simulink model "ImuCalibrator3Pass"  (R2018a)
settings: Solver=FixedStepDiscrete  StartTime=0.0  StopTime=inf  FixedStep=1/Fss  RelTol=1e-3
PreLoadFcn:
  | busDef
  | Fss = 1125;
  | Fss = 2100;
InitFcn:
  | modelDef = getModelDef(true);
undefined symbols (not defined in the file or in its folder): df, dw, Ggyr, Macc, Mgyr, numStates
libraries: simulink x15, vrlib x15, dspsigops x6, dspindex x6, dspinverses x6, dspstat3 x3, simulink_extras x3, dspmtrx3 x3, dspsrcs4 x3, dspmathops x3, dspswit3 x1
(part 4 of 4)

== matlab function ImuCalibrator3Pass/saveCalQuality ==
  data: fileReadError input; limits input; numStills input; firstPassCorrections input Bus: corrections; secondPassCorrections input Bus: corrections; thirdPassCorrections input Bus: corrections; calPass output
function calPass = saveCalQuality(fileReadError, limits, numStills, firstPassCorrections, secondPassCorrections, thirdPassCorrections)

fid = fopen('imuCalQuality.txt', 'w');
calPass = true;

if fileReadError
    calPass = false;
    fprintf(fid, 'FAIL :  imudata.txt file not read\n');
end

if numStills < 6
    calPass = false;
    fprintf(fid, 'FAIL : insufficient still times detected (possibly noisy sensor)\n');
end
fprintf(fid, 'Num stills over 5s duration: %d\n\n', int8(numStills));

% first pass corrections
fprintf(fid, '**********************  FIRST PASS ****************************\n');
gyroBiasLim = limits(1,1); %3*0.01;
gyroSfLim = limits(1,2);  %3*0.01;
gyroMaLim = limits(1,3);  %3*0.01;
accelBiasLim = limits(1,4);  %3*40*9.8/1000;
accelSfLim = limits(1,5);  %3*0.01;
accelMaLim = limits(1,6);  %3*0.01;
corrections = firstPassCorrections;
gyroBiases = [ corrections.dw(1) corrections.dw(2) corrections.dw(3)];
gyroSf = [corrections.Mgyr(1,1) corrections.Mgyr(2,2) corrections.Mgyr(3,3)];
gyroMa = [corrections.Mgyr(1,2) corrections.Mgyr(1,3) corrections.Mgyr(2,1) corrections.Mgyr(2,3) corrections.Mgyr(3,1) corrections.Mgyr(3,2)];
accelBiases = [ corrections.df(1) corrections.df(2) corrections.df(3)];
accelSf = [corrections.Macc(1,1) corrections.Macc(2,2) corrections.Macc(3,3)];
accelMa = [corrections.Macc(1,2) corrections.Macc(1,3) corrections.Macc(2,1) corrections.Macc(2,3) corrections.Macc(3,1) corrections.Macc(3,2)];



fprintf(fid, 'Gyro biases (deg/hr):\n');
rps2dph = 180/pi*3600;
calPass = calPass & printTriadResults(fid, gyroBiases*rps2dph, gyroBiasLim*rps2dph);

fprintf(fid, 'Gyro scale factors:\n');
calPass = calPass & printTriadResults(fid, gyroSf, gyroSfLim);

fprintf(fid, 'Gyro misalignments:\n');
calPass = calPass & printTriadResults(fid, gyroMa, gyroMaLim);

fprintf(fid, 'Accel biases (mg):\n');
mpss2mg = 1000/9.8;
calPass = calPass & printTriadResults(fid, accelBiases*mpss2mg, accelBiasLim*mpss2mg);

fprintf(fid, 'Accel scale factors:\n');
calPass = calPass & printTriadResults(fid, accelSf, accelSfLim);

fprintf(fid, 'Accel misalignments:\n');
calPass = calPass & printTriadResults(fid, accelMa, accelMaLim);



% second pass corrections
fprintf(fid, '**********************  SECOND PASS ****************************\n');
gyroBiasLim = limits(2,1);  %0.001;
gyroSfLim = limits(2,2);  %2e-3;
gyroMaLim = limits(2,3);  %2e-3;
accelBiasLim = limits(2,4);  %2 * 9.8/1000;
accelSfLim = limits(2,5);  %0.001;
accelMaLim = limits(2,6);  %0.003;
corrections = secondPassCorrections;
gyroBiases = [ corrections.dw(1) corrections.dw(2) corrections.dw(3)];
gyroSf = [corrections.Mgyr(1,1) corrections.Mgyr(2,2) corrections.Mgyr(3,3)];
gyroMa = [corrections.Mgyr(1,2) corrections.Mgyr(1,3) corrections.Mgyr(2,1) corrections.Mgyr(2,3) corrections.Mgyr(3,1) corrections.Mgyr(3,2)];
accelBiases = [ corrections.df(1) corrections.df(2) corrections.df(3)];
accelSf = [corrections.Macc(1,1) corrections.Macc(2,2) corrections.Macc(3,3)];
accelMa = [corrections.Macc(1,2) corrections.Macc(1,3) corrections.Macc(2,1) corrections.Macc(2,3) corrections.Macc(3,1) corrections.Macc(3,2)];

fprintf(fid, 'Gyro biases (deg/hr):\n');
rps2dph = 180/pi*3600;
calPass = calPass & printTriadResults(fid, gyroBiases*rps2dph, gyroBiasLim*rps2dph);

fprintf(fid, 'Gyro scale factors:\n');
calPass = calPass & printTriadResults(fid, gyroSf, gyroSfLim);

fprintf(fid, 'Gyro misalignments:\n');
calPass = calPass & printTriadResults(fid, gyroMa, gyroMaLim);

fprintf(fid, 'Accel biases (mg):\n');
mpss2mg = 1000/9.8;
calPass = calPass & printTriadResults(fid, accelBiases*mpss2mg, accelBiasLim*mpss2mg);

fprintf(fid, 'Accel scale factors:\n');
calPass = calPass & printTriadResults(fid, accelSf, accelSfLim);

fprintf(fid, 'Accel misalignments:\n');
calPass = calPass & printTriadResults(fid, accelMa, accelMaLim);



% third pass corrections
fprintf(fid, '**********************  THIRD PASS ****************************\n');
gyroBiasLim = limits(3,1); %3e-4;
gyroSfLim = limits(3,2); %2e-3;
gyroMaLim = limits(3,3); %2e-3;
accelBiasLim = limits(3,4); %0.3 * 9.8/1000;
accelSfLim = limits(3,5); %0.0003;
accelMaLim = limits(3,6); %0.0015;
corrections = thirdPassCorrections;
gyroBiases = [ corrections.dw(1) corrections.dw(2) corrections.dw(3)];
gyroSf = [corrections.Mgyr(1,1) corrections.Mgyr(2,2) corrections.Mgyr(3,3)];
gyroMa = [corrections.Mgyr(1,2) corrections.Mgyr(1,3) corrections.Mgyr(2,1) corrections.Mgyr(2,3) corrections.Mgyr(3,1) corrections.Mgyr(3,2)];
accelBiases = [ corrections.df(1) corrections.df(2) corrections.df(3)];
accelSf = [corrections.Macc(1,1) corrections.Macc(2,2) corrections.Macc(3,3)];
accelMa = [corrections.Macc(1,2) corrections.Macc(1,3) corrections.Macc(2,1) corrections.Macc(2,3) corrections.Macc(3,1) corrections.Macc(3,2)];

fprintf(fid, 'Gyro biases (deg/hr):\n');
rps2dph = 180/pi*3600;
calPass = calPass & printTriadResults(fid, gyroBiases*rps2dph, gyroBiasLim*rps2dph);

fprintf(fid, 'Gyro scale factors:\n');
calPass = calPass & printTriadResults(fid, gyroSf, gyroSfLim);

fprintf(fid, 'Gyro misalignments:\n');
calPass = calPass & printTriadResults(fid, gyroMa, gyroMaLim);

fprintf(fid, 'Accel biases (mg):\n');
mpss2mg = 1000/9.8;
calPass = calPass & printTriadResults(fid, accelBiases*mpss2mg, accelBiasLim*mpss2mg);

fprintf(fid, 'Accel scale factors:\n');
calPass = calPass & printTriadResults(fid, accelSf, accelSfLim);

fprintf(fid, 'Accel misalignments:\n');
calPass = calPass & printTriadResults(fid, accelMa, accelMaLim);






fclose(fid);

calPass = true;



function pass = printTriadResults(fid, values, limit)
for i=1:length(values)
    fprintf(fid, '%10.6f ', values(i)); 
end
fprintf(fid, '(limit %f) \n', limit);
pctLim = max(abs(values))/limit * 100;
if  pctLim <= 100 
    fprintf(fid, 'PASS (%4.1f %% of limit)\n\n', pctLim); pass = true;
else
    fprintf(fid, 'FAIL (%4.1f %% of limit)\n\n', pctLim);  pass = false;
end

== matlab function ImuCalibrator3Pass/MATLAB Function1 ==
  data: gyroCalBiases output; gyroCalMatrix output; dw input; Mgyr input; df input; Macc input; Ggyr input; accelCalBiases output; accelCalMatrix output; gyroGsensMatrix output
function [gyroCalBiases, gyroCalMatrix, accelCalBiases, accelCalMatrix,  gyroGsensMatrix] = updateCal(dw, Mgyr, df, Macc, Ggyr)

    

    gyroCalBiases =  (eye(3)+Mgyr)*dw;
    gyroGsensMatrix = (eye(3)+Mgyr)*Ggyr;
    gyroCalMatrix = inv(eye(3) + Mgyr);

    accelCalBiases =  df + Macc*df;
    accelCalMatrix =inv(eye(3) + Macc);

== matlab function ImuCalibrator3Pass/MATLAB Function2 ==
  data: gyroCalBiases output; gyroCalMatrix output; dw input; Mgyr input; df input; Macc input; Ggyr input; gyroCalBiases input; gyroCalMatrix input; accelCalBiases input; accelCalMatrix input; gyroGsensMatrix input; accelCalBiases output; accelCalMatrix output; gyroGsensMatrix output
function [gyroCalBiases, gyroCalMatrix, accelCalBiases, accelCalMatrix,  gyroGsensMatrix] = updateCal2(dw, Mgyr, df, Macc, Ggyr, gyroCalBiases, gyroCalMatrix, accelCalBiases, accelCalMatrix,  gyroGsensMatrix)

    gyroCalBiases = gyroCalBiases + (eye(3)+Mgyr)*dw;
    gyroGsensMatrix = gyroGsensMatrix + (eye(3)+Mgyr)*Ggyr;
    gyroCalMatrix = inv(eye(3) + Mgyr) * gyroCalMatrix;

    accelCalBiases = accelCalBiases + df + Macc*df;
    accelCalMatrix =inv(eye(3) + Macc) * accelCalMatrix;

== matlab function ImuCalibrator3Pass/firstPass/MATLAB Function1 ==
  data: datarow output; EOF output
function [datarow, EOF] = readLineAscii()

persistent data data2 nrows row

if isempty(data)
    % row format = # SeqID, DeviceID, timestamp (sec), gyroXYZ (rad/sec), accelXYZ (m/s^2), temperature (degC)
    coder.varsize('data', [500000, 10], [1 0]);  % ten columns,  up to 200k rows
    data = load('imudata.txt', '-ascii'); 
    
    validTimestamp = data(:,3) > 0.001;
    data2 = data(validTimestamp, [4 5 6 7 8 9 3]); % select just the useful columns and rows
    nrows = size(data2, 1);
    row = 2;  % skip the first row since we need delta-t's

end

datarow = data2(row,:)';
datarow(7) = data2(row,7) - data2(row-1,7); % calculate Delta-t

EOF = row >= nrows;
row = row + 1;

== matlab function ImuCalibrator3Pass/secondPass/AINS/INS/MATLAB Function2 ==
  data: Cbn input; Cbn_new output; w input; dt input
function Cbn_new = update_dcm(Cbn, w, dt)

% Update attitude according to TW p.312 approximated to sixth order

rot=w*dt;
rot_norm=norm(rot);
sr_a=1-(rot_norm^2/6)+(rot_norm^4/120);
sr_b=(1/2)-(rot_norm^2/24)+(rot_norm^4/720);
mx_a=eye(3)+sr_a*skew(rot)+sr_b*skew(rot)*skew(rot);

Cbn_new=Cbn*mx_a;


function res=skew(inp_vr)
res=[0 			-inp_vr(3)	inp_vr(2); ...
     inp_vr(3)	0			-inp_vr(1);...
	 -inp_vr(2)	inp_vr(1)	0];

== matlab function ImuCalibrator3Pass/secondPass/AINS/MATLAB Function ==
  data: w input; stilltime output; f input; Dt input; favgs output; wavgs output
function [stilltime, favgs, wavgs] = update_stilltime(w, f, Dt)

persistent stillt wavg favg stillcycles wsigmas fsigmas;

if isempty(wavg)
    stillt = 0;
    stillcycles = 0;
    wavg = w;
    favg = f;
    wsigmas = 0.02*[1;1;1];%%0.01*[1;1;1];
    fsigmas = 0.4*[1;1;1];%0.2*[1;1;1];
end

if all(abs(f-favg) < 3*fsigmas) && all(abs(w-wavg) < 3*wsigmas)  % increment the stilltimes
    stillt = stillt + Dt;
    stillcycles = stillcycles + 1;
%     % simple recursive mean (weighting all the samples equally):
%     wavg = ((stillcycles-1)*wavg + w)/stillcycles;
%     favg = ((stillcycles-1)*favg + f)/stillcycles;

%     % recursive mean with each sample weighted by the stillcycles when it came in:
%     wavg = ((stillcycles-1)*wavg + 2*w)/(stillcycles+1);
%     favg = ((stillcycles-1)*favg + 2*f)/(stillcycles+1);

    % start with stilltime weighting and switch back to simple recursive mean after 1 second to reduce noise:
    if stillt < 1
        wavg = ((stillcycles-1)*wavg + 2*w)/(stillcycles+1);
        favg = ((stillcycles-1)*favg + 2*f)/(stillcycles+1);
    else
        wavg = ((stillcycles-1)*wavg + w)/stillcycles;
        favg = ((stillcycles-1)*favg + f)/stillcycles;
    end        
else  %reset stilltime
    stillt = 0;
    stillcycles = 0;
    wavg = w;
    favg = f;
end    

stilltime = stillt;
favgs = favg;
wavgs = wavg;

== matlab function ImuCalibrator3Pass/secondPass/AINS/compass meas update/MATLAB Function1 ==
  data: S output; P input; K output; H input; R input
function [S,K] = calcKalmanGain(P, H, R)

PHT = P*H';
S = H*PHT + R;
K = PHT/S;

== matlab function ImuCalibrator3Pass/secondPass/AINS/compass meas update/MATLAB Function3 ==
  data: P input; Pplus output; K input; H input; R input; IminKH output
function [Pplus, IminKH] = josephCovarianceUpdate(P, K, H, R)

IminKH = eye(size(P)) - K*H;
Pplus = IminKH*P*IminKH' + K*R*K';

== matlab function ImuCalibrator3Pass/secondPass/AINS/compass meas update/update the Cbn with the errors/MATLAB Function ==
  data: inp_vr input; res output
function res=skew(inp_vr)
res=[0 			-inp_vr(3)	inp_vr(2); ...
     inp_vr(3)	0			-inp_vr(1);...
	 -inp_vr(2)	inp_vr(1)	0];

== matlab function ImuCalibrator3Pass/firstPass/AINS/gravity meas update/MATLAB Function2 ==
  data: inp_vr input; res output
function res=skew(inp_vr)
res=[0 			-inp_vr(3)	inp_vr(2); ...
     inp_vr(3)	0			-inp_vr(1);...
	 -inp_vr(2)	inp_vr(1)	0];

== matlab function ImuCalibrator3Pass/firstPass/AINS/compass meas update/MATLAB Function1 ==
  data: S output; P input; K output; H input; R input
function [S,K] = calcKalmanGain(P, H, R)

PHT = P*H';
S = H*PHT + R;
K = PHT/S;

== matlab function ImuCalibrator3Pass/secondPass/AINS/gravity meas update/MATLAB Function1 ==
  data: S output; P input; K output; H input; R input
function [S,K] = calcKalmanGain(P, H, R)

PHT = P*H';
S = H*PHT + R;
K = PHT/S;

== matlab function ImuCalibrator3Pass/secondPass/AINS/gravity meas update/MATLAB Function2 ==
  data: inp_vr input; res output
function res=skew(inp_vr)
res=[0 			-inp_vr(3)	inp_vr(2); ...
     inp_vr(3)	0			-inp_vr(1);...
	 -inp_vr(2)	inp_vr(1)	0];

== matlab function ImuCalibrator3Pass/secondPass/AINS/gravity meas update/MATLAB Function3 ==
  data: P input; Pplus output; K input; H input; R input; IminKH output
function [Pplus, IminKH] = josephCovarianceUpdate(P, K, H, R)

IminKH = eye(size(P)) - K*H;
Pplus = IminKH*P*IminKH' + K*R*K';

== matlab function ImuCalibrator3Pass/secondPass/AINS/gravity meas update/update the Cbn and b_g with the errors/MATLAB Function ==
  data: inp_vr input; res output
function res=skew(inp_vr)
res=[0 			-inp_vr(3)	inp_vr(2); ...
     inp_vr(3)	0			-inp_vr(1);...
	 -inp_vr(2)	inp_vr(1)	0];

== matlab function ImuCalibrator3Pass/secondPass/AINS/initialize states and covariances/set P/MATLAB Function1 ==
  data: initialRotUncert input; initialPosUncert input; initialVelUncert input; P0 output size=[modelDef.numStates, modelDef.numStates]; modelDef parameter; imuPar parameter
function P0  = calculate_P0(initialRotUncert, initialPosUncert, initialVelUncert, modelDef, imuPar)

% order of the states:
% 1:3   phi
% 4:6   dw
% 7:9   dr
% 10:12 dv
% 13:15 df  (if modelDef.trackAccelBiases)
% 16:24 dM_gyro in column-major order (if modelDef.trackGyroSfma)
% 25:33 dM_accel in column-major order (if modelDef.trackAccelSfma)
% 34:42 dG_gyro in column-major order (if modelDef.trackGyroGsens)

P0 = zeros(modelDef.numStates, modelDef.numStates);

P0(1:3, 1:3) = diag(initialRotUncert.^2);
P0(4:6, 4:6) = eye(3)*(imuPar.gyroBiasUncert.^2);
P0(7:9, 7:9) = diag(initialPosUncert.^2);
P0(10:12, 10:12) = diag(initialVelUncert.^2);


if modelDef.trackAccelBiases
    P0(13:15, 13:15) = eye(3)*(imuPar.accelBiasUncert.^2);
end

if modelDef.trackGyroSfma  
    vec9 = ones(9,1)*imuPar.gyroAlignUncert^2;
    vec9([1 5 9]) = imuPar.gyroScaleUncert^2;
    P0(16:24, 16:24) = diag(vec9);
end

if modelDef.trackAccelSfma  % propagate dM_accel to dv
    vec9 = ones(9,1)*imuPar.accelAlignUncert^2;
    vec9([1 5 9]) = imuPar.accelScaleUncert^2;
    if modelDef.accelDefinesExtrinsics
        vec9([4 7]) = 0.0001^2; % x accel has no misalignment so picks up no component of y or z accelerations
        vec9(8) = 0.0001^2;  % y accel has no tilt out of xy plane, so picks up no component of z acceleration
    end
    P0(25:33, 25:33) = diag(vec9);
end

if modelDef.trackGyroGsens
    vec9 = ones(9,1)*imuPar.gyroGsensUncert^2;
    P0(34:42, 34:42) = diag(vec9);
end

== matlab function ImuCalibrator3Pass/firstPass/AINS/compass meas update/MATLAB Function3 ==
  data: P input; Pplus output; K input; H input; R input; IminKH output
function [Pplus, IminKH] = josephCovarianceUpdate(P, K, H, R)

IminKH = eye(size(P)) - K*H;
Pplus = IminKH*P*IminKH' + K*R*K';

== matlab function ImuCalibrator3Pass/secondPass/AINS/report output/MATLAB Function1 ==
  data: Cbn input; quat output size=[4,1]
function quat=dcm2quat(Cbn)

%dcm (Cba) to quaternion (qba)
%Cba:B to A transformation matrix
%qba:B to A quaternion

%Implementation of savage(3-47)


tr=Cbn(1,1)+Cbn(2,2)+Cbn(3,3);
Pa=1+tr;
Pb=1+2*Cbn(1,1)-tr;
Pc=1+2*Cbn(2,2)-tr;
Pd=1+2*Cbn(3,3)-tr;

quat=zeros(4,1);
if (Pa>=Pb && Pa>=Pc && Pa>=Pd)
    quat(1)=0.5*sqrt(Pa);
    quat(2)=(Cbn(3,2)-Cbn(2,3))/4/quat(1);
    quat(3)=(Cbn(1,3)-Cbn(3,1))/4/quat(1);
    quat(4)=(Cbn(2,1)-Cbn(1,2))/4/quat(1);
elseif (Pb>=Pc && Pb>=Pd)
    quat(2)=0.5*sqrt(Pb);
    quat(3)=(Cbn(2,1)+Cbn(1,2))/4/quat(2);
    quat(4)=(Cbn(1,3)+Cbn(3,1))/4/quat(2);
    quat(1)=(Cbn(3,2)-Cbn(2,3))/4/quat(2);
elseif (Pc>=Pd)
    quat(3)=0.5*sqrt(Pc);
    quat(4)=(Cbn(3,2)+Cbn(2,3))/4/quat(3);
    quat(1)=(Cbn(1,3)-Cbn(3,1))/4/quat(3);
    quat(2)=(Cbn(2,1)+Cbn(1,2))/4/quat(3);
else
    quat(4)=0.5*sqrt(Pd);
    quat(1)=(Cbn(2,1)-Cbn(1,2))/4/quat(4);
    quat(2)=(Cbn(1,3)+Cbn(3,1))/4/quat(4);
    quat(3)=(Cbn(3,2)+Cbn(2,3))/4/quat(4);
end

if (quat(1)<=0)
    quat=-quat;
end

== matlab function ImuCalibrator3Pass/secondPass/AINS/report output/MATLAB Function3 ==
  data: Cbn input; eul output size=[3,1]
function eul = dcm2euler(Cbn)

%DCM is Cbn (transforms vectors from b to n)
%eul defined as zyx sequence (yaw,pitch,roll),  but listed in
%roll,pitch,yaw order


pitch=asin(-Cbn(3,1));  %pitch is assumed to be [-pi pi]. singular at pi. use ad-hoc methods to remedy this deficiency
roll=atan2(Cbn(3,2), Cbn(3,3));
heading = atan2(Cbn(2,1), Cbn(1,1));
eul=[roll;pitch;heading];

== matlab function ImuCalibrator3Pass/firstPass/AINS/compass meas update/update the Cbn with the errors/MATLAB Function ==
  data: inp_vr input; res output
function res=skew(inp_vr)
res=[0 			-inp_vr(3)	inp_vr(2); ...
     inp_vr(3)	0			-inp_vr(1);...
	 -inp_vr(2)	inp_vr(1)	0];

== matlab function ImuCalibrator3Pass/secondPass/AINS/time update/MATLAB Function ==
  data: omega input; Q output size=[modelDef.numStates, modelDef.numStates]; f_ib input; Dt input; Cbn input; modelDef parameter; imuPar parameter
function Q  = calculate_Q(omega, f_ib, Dt, Cbn, modelDef, imuPar)

% order of the states:
% 1:3   phi
% 4:6   dw
% 7:9   dr
% 10:12 dv
% 13:15 df  (if modelDef.trackAccelBiases)
% 16:24 dM_gyro in column-major order (if modelDef.trackGyroSfma)
% 25:33 dM_accel in column-major order (if modelDef.trackAccelSfma)

Q = zeros(modelDef.numStates, modelDef.numStates);

omega = reshape(omega,3,1); 
f_ib = reshape(f_ib, 3,1);

Qphi = diag((imuPar.gyroArwRadPerRtSec^2)*[Dt Dt Dt]);  
Qdw = diag((imuPar.gyroBrwRadPerSecPerRtSec^2)*[Dt Dt Dt]);
Qdv = diag((imuPar.accelVrwMetersPerSecPerRtSec^2)*[Dt Dt Dt]);
Qdf = diag((imuPar.accelBrwMetersPerSec2PerRtSec^2)*[Dt Dt Dt]);


%bump up Q for unmodelled states
if ~modelDef.trackGyroSfma % gyro scale factor and misalignment not tracked
   gyroSfSigmaBod = imuPar.gyroScaleUncert*omega;
   gyroMaSigmaBod = imuPar.gyroAlignUncert*sqrt(omega'*omega*[1 1 1]-omega'.*omega');   
   QgyroMa = Cbn*diag(gyroMaSigmaBod.^2)*Cbn'*Dt; 
   QgyroSf = Cbn*diag(gyroSfSigmaBod.^2)*Cbn'*Dt; 
   Qphi = Qphi + QgyroMa + QgyroSf;   
end

if ~modelDef.trackGyroGsens %  gyro g sensitivity not tracked 
   gGsensSigmaBod = imuPar.gyroGsensUncert*sqrt(f_ib'*f_ib*[1 1 1]-f_ib'.*f_ib');   
   QgGsens = Cbn*diag(gGsensSigmaBod.^2)*Cbn'*Dt; 
   Qphi = Qphi + QgGsens;   
end

if ~modelDef.trackAccelSfma  % accel scale factor and misalignment not tracked
   accelSfSigmaBod = imuPar.accelScaleUncert*f_ib;
   accelMaSigmaBod = imuPar.accelAlignUncert*sqrt(f_ib'*f_ib*[1 1 1]-f_ib'.*f_ib');   
   QaccelMa = Cbn*diag(accelMaSigmaBod.^2)*Cbn'*Dt; 
   QaccelSf = Cbn*diag(accelSfSigmaBod.^2)*Cbn'*Dt; 
   Qdv = Qdv + QaccelMa + QaccelSf;   
end

Q(1:3, 1:3) = Qphi;
Q(4:6, 4:6) = Qdw;
Q(10:12, 10:12) = Qdv;
Q(13:15, 13:15) = Qdf;

== matlab function ImuCalibrator3Pass/secondPass/AINS/time update/MATLAB Function1 ==
  data: imuPar output Bus: imuPar
function imuPar = imuPar

imuPar.gyroArwDegPerRtHr = 0.25;
imuPar.gyroArwRadPerRtSec = imuPar.gyroArwDegPerRtHr * pi/180/60;
imuPar.gyroBrwDegPerHrPerRtHr = 0;
imuPar.gyroBrwRadPerSecPerRtSec = imuPar.gyroBrwDegPerHrPerRtHr * pi/180/3600/60;
imuPar.gyroScaleUncertainty = 0.001;
imuPar.gyroAlignUncertainty = 0.01;
imuPar.gyroGsensUncertainty = 0.001;

== matlab function ImuCalibrator3Pass/secondPass/AINS/time update/MATLAB Function2 ==
  settings: updateMethod=DISCRETE  sampleTime=inf
  data: modelDef output Bus: modelDef; numStates input
function modelDef = modelDef(numStates)

modelDef.trackAccelBiases = true;
modelDef.trackAccelSfma = true;
modelDef.trackGyroSfma = true;
modelDef.trackGyroGsens = false;

modelDef.numStates = numStates;

== matlab function ImuCalibrator3Pass/secondPass/AINS/time update/MATLAB Function3 ==
  data: omega input; Phi output size=[modelDef.numStates, modelDef.numStates]; fbod input; Dt input; Cbn input; modelDef parameter
function Phi  = calculate_Phi(omega, fbod, Dt, Cbn, modelDef)

% order of the states:
% 1:3   phi
% 4:6   dw
% 7:9   dr
% 10:12 dv
% 13:15 df  (if modelDef.trackAccelBiases)
% 16:24 dM_gyro in column-major order (if modelDef.trackGyroSfma)
% 25:33 dM_accel in column-major order (if modelDef.trackAccelSfma)
% 34:42 dG_gyro in column-major order (if modelDef.trackGyroGsens)

Phi = eye(modelDef.numStates);

DtC = Dt*Cbn;

Phi(1:3,4:6) = -DtC;  % propagate dw to phi
Phi(7:9, 10:12) = Dt*eye(3);  % propagate dv to dr
Phi(10:12, 1:3) = Dt*skew(Cbn*fbod);  % propagate phi to dv

if modelDef.trackAccelBiases
    Phi(10:12, 13:15) = DtC;   % propagate df to dv
end

if modelDef.trackGyroSfma  % propagate dM_gyro to phi
    Phi(1:3, 16:18) = -DtC*omega(1);
    Phi(1:3, 19:21) = -DtC*omega(2);
    Phi(1:3, 22:24) = -DtC*omega(3);
end

if modelDef.trackAccelSfma  % propagate dM_accel to dv
    Phi(10:12, 25:27) = DtC*fbod(1);
    Phi(10:12, 28:30) = DtC*fbod(2);
    Phi(10:12, 31:33) = DtC*fbod(3);
end

if modelDef.trackGyroGsens  % propagate dG_gyro to phi
    Phi(1:3, 34:36) = -DtC*fbod(1);
    Phi(1:3, 37:39) = -DtC*fbod(2);
    Phi(1:3, 40:42) = -DtC*fbod(3);
end


function res=skew(inp_vr)
res=[0 			-inp_vr(3)	inp_vr(2); ...
     inp_vr(3)	0			-inp_vr(1);...
	 -inp_vr(2)	inp_vr(1)	0];

== matlab function ImuCalibrator3Pass/secondPass/AINS/zero velocity update/MATLAB Function1 ==
  data: S output; P input; K output; H input; R input
function [S,K] = calcKalmanGain(P, H, R)

PHT = P*H';
S = H*PHT + R;
K = PHT/S;

== matlab function ImuCalibrator3Pass/secondPass/AINS/zero velocity update/MATLAB Function3 ==
  data: P input; Pplus output; K input; H input; R input; IminKH output
function [Pplus, IminKH] = josephCovarianceUpdate(P, K, H, R)

IminKH = eye(size(P)) - K*H;
Pplus = IminKH*P*IminKH' + K*R*K';

== matlab function ImuCalibrator3Pass/secondPass/AINS/zero velocity update/update the underlying states/MATLAB Function ==
  data: inp_vr input; res output
function res=skew(inp_vr)
res=[0 			-inp_vr(3)	inp_vr(2); ...
     inp_vr(3)	0			-inp_vr(1);...
	 -inp_vr(2)	inp_vr(1)	0];

== matlab function ImuCalibrator3Pass/secondPass/printTime/MATLAB Function ==
  data: u input
function  printTime(u)
%#codegen

% using fileId = 1  only generates a printf in the generated code
% fileId = 2 also causes prints in the matlab console

fprintf(2, "\r 2nd pass: %f sec", u);

== matlab function ImuCalibrator3Pass/thirdPass/AINS/INS/MATLAB Function2 ==
  data: Cbn input; Cbn_new output; w input; dt input
function Cbn_new = update_dcm(Cbn, w, dt)

% Update attitude according to TW p.312 approximated to sixth order

rot=w*dt;
rot_norm=norm(rot);
sr_a=1-(rot_norm^2/6)+(rot_norm^4/120);
sr_b=(1/2)-(rot_norm^2/24)+(rot_norm^4/720);
mx_a=eye(3)+sr_a*skew(rot)+sr_b*skew(rot)*skew(rot);

Cbn_new=Cbn*mx_a;


function res=skew(inp_vr)
res=[0 			-inp_vr(3)	inp_vr(2); ...
     inp_vr(3)	0			-inp_vr(1);...
	 -inp_vr(2)	inp_vr(1)	0];

== matlab function ImuCalibrator3Pass/thirdPass/AINS/MATLAB Function ==
  data: w input; stilltime output; f input; Dt input; favgs output; wavgs output
function [stilltime, favgs, wavgs] = update_stilltime(w, f, Dt)

persistent stillt wavg favg stillcycles wsigmas fsigmas;

if isempty(wavg)
    stillt = 0;
    stillcycles = 0;
    wavg = w;
    favg = f;
    wsigmas = 0.02*[1;1;1];%%0.01*[1;1;1];
    fsigmas = 0.4*[1;1;1];%0.2*[1;1;1];
end

if all(abs(f-favg) < 3*fsigmas) && all(abs(w-wavg) < 3*wsigmas)  % increment the stilltimes
    stillt = stillt + Dt;
    stillcycles = stillcycles + 1;
%     % simple recursive mean (weighting all the samples equally):
%     wavg = ((stillcycles-1)*wavg + w)/stillcycles;
%     favg = ((stillcycles-1)*favg + f)/stillcycles;

%     % recursive mean with each sample weighted by the stillcycles when it came in:
%     wavg = ((stillcycles-1)*wavg + 2*w)/(stillcycles+1);
%     favg = ((stillcycles-1)*favg + 2*f)/(stillcycles+1);

    % start with stilltime weighting and switch back to simple recursive mean after 1 second to reduce noise:
    if stillt < 1
        wavg = ((stillcycles-1)*wavg + 2*w)/(stillcycles+1);
        favg = ((stillcycles-1)*favg + 2*f)/(stillcycles+1);
    else
        wavg = ((stillcycles-1)*wavg + w)/stillcycles;
        favg = ((stillcycles-1)*favg + f)/stillcycles;
    end        
else  %reset stilltime
    stillt = 0;
    stillcycles = 0;
    wavg = w;
    favg = f;
end    

stilltime = stillt;
favgs = favg;
wavgs = wavg;

== matlab function ImuCalibrator3Pass/thirdPass/AINS/compass meas update/MATLAB Function1 ==
  data: S output; P input; K output; H input; R input
function [S,K] = calcKalmanGain(P, H, R)

PHT = P*H';
S = H*PHT + R;
K = PHT/S;

== matlab function ImuCalibrator3Pass/thirdPass/AINS/compass meas update/MATLAB Function3 ==
  data: P input; Pplus output; K input; H input; R input; IminKH output
function [Pplus, IminKH] = josephCovarianceUpdate(P, K, H, R)

IminKH = eye(size(P)) - K*H;
Pplus = IminKH*P*IminKH' + K*R*K';

== matlab function ImuCalibrator3Pass/thirdPass/AINS/compass meas update/update the Cbn with the errors/MATLAB Function ==
  data: inp_vr input; res output
function res=skew(inp_vr)
res=[0 			-inp_vr(3)	inp_vr(2); ...
     inp_vr(3)	0			-inp_vr(1);...
	 -inp_vr(2)	inp_vr(1)	0];

== matlab function ImuCalibrator3Pass/thirdPass/AINS/gravity meas update/MATLAB Function1 ==
  data: S output; P input; K output; H input; R input
function [S,K] = calcKalmanGain(P, H, R)

PHT = P*H';
S = H*PHT + R;
K = PHT/S;

== matlab function ImuCalibrator3Pass/thirdPass/AINS/gravity meas update/MATLAB Function2 ==
  data: inp_vr input; res output
function res=skew(inp_vr)
res=[0 			-inp_vr(3)	inp_vr(2); ...
     inp_vr(3)	0			-inp_vr(1);...
	 -inp_vr(2)	inp_vr(1)	0];

== matlab function ImuCalibrator3Pass/thirdPass/AINS/gravity meas update/MATLAB Function3 ==
  data: P input; Pplus output; K input; H input; R input; IminKH output
function [Pplus, IminKH] = josephCovarianceUpdate(P, K, H, R)

IminKH = eye(size(P)) - K*H;
Pplus = IminKH*P*IminKH' + K*R*K';

== matlab function ImuCalibrator3Pass/thirdPass/AINS/gravity meas update/update the Cbn and b_g with the errors/MATLAB Function ==
  data: inp_vr input; res output
function res=skew(inp_vr)
res=[0 			-inp_vr(3)	inp_vr(2); ...
     inp_vr(3)	0			-inp_vr(1);...
	 -inp_vr(2)	inp_vr(1)	0];

== matlab function ImuCalibrator3Pass/thirdPass/AINS/initialize states and covariances/set P/MATLAB Function1 ==
  data: initialRotUncert input; initialPosUncert input; initialVelUncert input; P0 output size=[modelDef.numStates, modelDef.numStates]; modelDef parameter; imuPar parameter
function P0  = calculate_P0(initialRotUncert, initialPosUncert, initialVelUncert, modelDef, imuPar)

% order of the states:
% 1:3   phi
% 4:6   dw
% 7:9   dr
% 10:12 dv
% 13:15 df  (if modelDef.trackAccelBiases)
% 16:24 dM_gyro in column-major order (if modelDef.trackGyroSfma)
% 25:33 dM_accel in column-major order (if modelDef.trackAccelSfma)
% 34:42 dG_gyro in column-major order (if modelDef.trackGyroGsens)

P0 = zeros(modelDef.numStates, modelDef.numStates);

P0(1:3, 1:3) = diag(initialRotUncert.^2);
P0(4:6, 4:6) = eye(3)*(imuPar.gyroBiasUncert.^2);
P0(7:9, 7:9) = diag(initialPosUncert.^2);
P0(10:12, 10:12) = diag(initialVelUncert.^2);


if modelDef.trackAccelBiases
    P0(13:15, 13:15) = eye(3)*(imuPar.accelBiasUncert.^2);
end

if modelDef.trackGyroSfma  
    vec9 = ones(9,1)*imuPar.gyroAlignUncert^2;
    vec9([1 5 9]) = imuPar.gyroScaleUncert^2;
    P0(16:24, 16:24) = diag(vec9);
end

if modelDef.trackAccelSfma  % propagate dM_accel to dv
    vec9 = ones(9,1)*imuPar.accelAlignUncert^2;
    vec9([1 5 9]) = imuPar.accelScaleUncert^2;
    if modelDef.accelDefinesExtrinsics
        vec9([4 7]) = 0.0001^2; % x accel has no misalignment so picks up no component of y or z accelerations
        vec9(8) = 0.0001^2;  % y accel has no tilt out of xy plane, so picks up no component of z acceleration
    end
    P0(25:33, 25:33) = diag(vec9);
end

if modelDef.trackGyroGsens
    vec9 = ones(9,1)*imuPar.gyroGsensUncert^2;
    P0(34:42, 34:42) = diag(vec9);
end

== matlab function ImuCalibrator3Pass/thirdPass/AINS/report output/MATLAB Function1 ==
  data: Cbn input; quat output size=[4,1]
function quat=dcm2quat(Cbn)

%dcm (Cba) to quaternion (qba)
%Cba:B to A transformation matrix
%qba:B to A quaternion

%Implementation of savage(3-47)


tr=Cbn(1,1)+Cbn(2,2)+Cbn(3,3);
Pa=1+tr;
Pb=1+2*Cbn(1,1)-tr;
Pc=1+2*Cbn(2,2)-tr;
Pd=1+2*Cbn(3,3)-tr;

quat=zeros(4,1);
if (Pa>=Pb && Pa>=Pc && Pa>=Pd)
    quat(1)=0.5*sqrt(Pa);
    quat(2)=(Cbn(3,2)-Cbn(2,3))/4/quat(1);
    quat(3)=(Cbn(1,3)-Cbn(3,1))/4/quat(1);
    quat(4)=(Cbn(2,1)-Cbn(1,2))/4/quat(1);
elseif (Pb>=Pc && Pb>=Pd)
    quat(2)=0.5*sqrt(Pb);
    quat(3)=(Cbn(2,1)+Cbn(1,2))/4/quat(2);
    quat(4)=(Cbn(1,3)+Cbn(3,1))/4/quat(2);
    quat(1)=(Cbn(3,2)-Cbn(2,3))/4/quat(2);
elseif (Pc>=Pd)
    quat(3)=0.5*sqrt(Pc);
    quat(4)=(Cbn(3,2)+Cbn(2,3))/4/quat(3);
    quat(1)=(Cbn(1,3)-Cbn(3,1))/4/quat(3);
    quat(2)=(Cbn(2,1)+Cbn(1,2))/4/quat(3);
else
    quat(4)=0.5*sqrt(Pd);
    quat(1)=(Cbn(2,1)-Cbn(1,2))/4/quat(4);
    quat(2)=(Cbn(1,3)+Cbn(3,1))/4/quat(4);
    quat(3)=(Cbn(3,2)+Cbn(2,3))/4/quat(4);
end

if (quat(1)<=0)
    quat=-quat;
end

== matlab function ImuCalibrator3Pass/thirdPass/AINS/report output/MATLAB Function3 ==
  data: Cbn input; eul output size=[3,1]
function eul = dcm2euler(Cbn)

%DCM is Cbn (transforms vectors from b to n)
%eul defined as zyx sequence (yaw,pitch,roll),  but listed in
%roll,pitch,yaw order


pitch=asin(-Cbn(3,1));  %pitch is assumed to be [-pi pi]. singular at pi. use ad-hoc methods to remedy this deficiency
roll=atan2(Cbn(3,2), Cbn(3,3));
heading = atan2(Cbn(2,1), Cbn(1,1));
eul=[roll;pitch;heading];

== matlab function ImuCalibrator3Pass/thirdPass/AINS/time update/MATLAB Function ==
  data: omega input; Q output size=[modelDef.numStates, modelDef.numStates]; f_ib input; Dt input; Cbn input; modelDef parameter; imuPar parameter
function Q  = calculate_Q(omega, f_ib, Dt, Cbn, modelDef, imuPar)

% order of the states:
% 1:3   phi
% 4:6   dw
% 7:9   dr
% 10:12 dv
% 13:15 df  (if modelDef.trackAccelBiases)
% 16:24 dM_gyro in column-major order (if modelDef.trackGyroSfma)
% 25:33 dM_accel in column-major order (if modelDef.trackAccelSfma)

Q = zeros(modelDef.numStates, modelDef.numStates);

omega = reshape(omega,3,1); 
f_ib = reshape(f_ib, 3,1);

Qphi = diag((imuPar.gyroArwRadPerRtSec^2)*[Dt Dt Dt]);  
Qdw = diag((imuPar.gyroBrwRadPerSecPerRtSec^2)*[Dt Dt Dt]);
Qdv = diag((imuPar.accelVrwMetersPerSecPerRtSec^2)*[Dt Dt Dt]);
Qdf = diag((imuPar.accelBrwMetersPerSec2PerRtSec^2)*[Dt Dt Dt]);


%bump up Q for unmodelled states
if ~modelDef.trackGyroSfma % gyro scale factor and misalignment not tracked
   gyroSfSigmaBod = imuPar.gyroScaleUncert*omega;
   gyroMaSigmaBod = imuPar.gyroAlignUncert*sqrt(omega'*omega*[1 1 1]-omega'.*omega');   
   QgyroMa = Cbn*diag(gyroMaSigmaBod.^2)*Cbn'*Dt; 
   QgyroSf = Cbn*diag(gyroSfSigmaBod.^2)*Cbn'*Dt; 
   Qphi = Qphi + QgyroMa + QgyroSf;   
end

if ~modelDef.trackGyroGsens %  gyro g sensitivity not tracked 
   gGsensSigmaBod = imuPar.gyroGsensUncert*sqrt(f_ib'*f_ib*[1 1 1]-f_ib'.*f_ib');   
   QgGsens = Cbn*diag(gGsensSigmaBod.^2)*Cbn'*Dt; 
   Qphi = Qphi + QgGsens;   
end

if ~modelDef.trackAccelSfma  % accel scale factor and misalignment not tracked
   accelSfSigmaBod = imuPar.accelScaleUncert*f_ib;
   accelMaSigmaBod = imuPar.accelAlignUncert*sqrt(f_ib'*f_ib*[1 1 1]-f_ib'.*f_ib');   
   QaccelMa = Cbn*diag(accelMaSigmaBod.^2)*Cbn'*Dt; 
   QaccelSf = Cbn*diag(accelSfSigmaBod.^2)*Cbn'*Dt; 
   Qdv = Qdv + QaccelMa + QaccelSf;   
end

Q(1:3, 1:3) = Qphi;
Q(4:6, 4:6) = Qdw;
Q(10:12, 10:12) = Qdv;
Q(13:15, 13:15) = Qdf;

== matlab function ImuCalibrator3Pass/thirdPass/AINS/time update/MATLAB Function1 ==
  data: imuPar output Bus: imuPar
function imuPar = imuPar

imuPar.gyroArwDegPerRtHr = 0.25;
imuPar.gyroArwRadPerRtSec = imuPar.gyroArwDegPerRtHr * pi/180/60;
imuPar.gyroBrwDegPerHrPerRtHr = 0;
imuPar.gyroBrwRadPerSecPerRtSec = imuPar.gyroBrwDegPerHrPerRtHr * pi/180/3600/60;
imuPar.gyroScaleUncertainty = 0.001;
imuPar.gyroAlignUncertainty = 0.01;
imuPar.gyroGsensUncertainty = 0.001;

== matlab function ImuCalibrator3Pass/thirdPass/AINS/time update/MATLAB Function2 ==
  settings: updateMethod=DISCRETE  sampleTime=inf
  data: modelDef output Bus: modelDef; numStates input
function modelDef = modelDef(numStates)

modelDef.trackAccelBiases = true;
modelDef.trackAccelSfma = true;
modelDef.trackGyroSfma = true;
modelDef.trackGyroGsens = false;

modelDef.numStates = numStates;

== matlab function ImuCalibrator3Pass/thirdPass/AINS/time update/MATLAB Function3 ==
  data: omega input; Phi output size=[modelDef.numStates, modelDef.numStates]; fbod input; Dt input; Cbn input; modelDef parameter
function Phi  = calculate_Phi(omega, fbod, Dt, Cbn, modelDef)

% order of the states:
% 1:3   phi
% 4:6   dw
% 7:9   dr
% 10:12 dv
% 13:15 df  (if modelDef.trackAccelBiases)
% 16:24 dM_gyro in column-major order (if modelDef.trackGyroSfma)
% 25:33 dM_accel in column-major order (if modelDef.trackAccelSfma)
% 34:42 dG_gyro in column-major order (if modelDef.trackGyroGsens)

Phi = eye(modelDef.numStates);

DtC = Dt*Cbn;

Phi(1:3,4:6) = -DtC;  % propagate dw to phi
Phi(7:9, 10:12) = Dt*eye(3);  % propagate dv to dr
Phi(10:12, 1:3) = Dt*skew(Cbn*fbod);  % propagate phi to dv

if modelDef.trackAccelBiases
    Phi(10:12, 13:15) = DtC;   % propagate df to dv
end

if modelDef.trackGyroSfma  % propagate dM_gyro to phi
    Phi(1:3, 16:18) = -DtC*omega(1);
    Phi(1:3, 19:21) = -DtC*omega(2);
    Phi(1:3, 22:24) = -DtC*omega(3);
end

if modelDef.trackAccelSfma  % propagate dM_accel to dv
    Phi(10:12, 25:27) = DtC*fbod(1);
    Phi(10:12, 28:30) = DtC*fbod(2);
    Phi(10:12, 31:33) = DtC*fbod(3);
end

if modelDef.trackGyroGsens  % propagate dG_gyro to phi
    Phi(1:3, 34:36) = -DtC*fbod(1);
    Phi(1:3, 37:39) = -DtC*fbod(2);
    Phi(1:3, 40:42) = -DtC*fbod(3);
end

function res=skew(inp_vr)
res=[0 			-inp_vr(3)	inp_vr(2); ...
     inp_vr(3)	0			-inp_vr(1);...
	 -inp_vr(2)	inp_vr(1)	0];

== matlab function ImuCalibrator3Pass/thirdPass/AINS/zero velocity update/MATLAB Function1 ==
  data: S output; P input; K output; H input; R input
function [S,K] = calcKalmanGain(P, H, R)

PHT = P*H';
S = H*PHT + R;
K = PHT/S;

== matlab function ImuCalibrator3Pass/thirdPass/AINS/zero velocity update/MATLAB Function3 ==
  data: P input; Pplus output; K input; H input; R input; IminKH output
function [Pplus, IminKH] = josephCovarianceUpdate(P, K, H, R)

IminKH = eye(size(P)) - K*H;
Pplus = IminKH*P*IminKH' + K*R*K';

== matlab function ImuCalibrator3Pass/thirdPass/AINS/zero velocity update/update the underlying states/MATLAB Function ==
  data: inp_vr input; res output
function res=skew(inp_vr)
res=[0 			-inp_vr(3)	inp_vr(2); ...
     inp_vr(3)	0			-inp_vr(1);...
	 -inp_vr(2)	inp_vr(1)	0];

== matlab function ImuCalibrator3Pass/thirdPass/printTime/MATLAB Function ==
  data: u input
function  printTime(u)
%#codegen

% using fileId = 1  only generates a printf in the generated code
% fileId = 2 also causes prints in the matlab console

fprintf(2, "\r 3rd pass: %f sec", u);

== matlab function ImuCalibrator3Pass/MATLAB Function3 ==
  data: calQuality input; gyroCalBiases input; done output; gyroCalMatrix input; accelCalBiases input; accelCalMatrix input; SensorTypeIdentifier input int32; filename input
function done = saveCal( calQuality, gyroCalBiases, gyroCalMatrix, accelCalBiases, accelCalMatrix, SensorTypeIdentifier, filename)

fname = char(filename);
fname2 = convertCharsToStrings(fname);
fid = fopen(fname2, 'w');


%  TODO:  perhaps the Rid could be automatically selected based on
%  SensorTypeIdentifier if we used different STIs for different boards?
Rid = [1 0 0; 0 0 1; 0 -1 0]; %LMVP & Rigel w/ break-out board
%Rid = [-1 0 0; 0 0 -1; 0 -1 0];  % Rigel with dead-bug-IMU nominal rotation from imu axes to device axes (x left, y forward, z down)

% accel block first:
cal3x4 = Rid*[accelCalMatrix -accelCalMatrix*accelCalBiases];
vec = reshape(cal3x4, 12, 1); % JSON file stores the cal3x4 elements in column-wide order:

fprintf(fid, '{\n');
fprintf(fid, '  "accelerometer": {\n');
fprintf(fid, '    "%d": [\n', SensorTypeIdentifier);
for i=1:12
    fprintf(fid, '      %8.6f,\n', vec(i) );
end
fprintf(fid, '    ]\n');
fprintf(fid, '  },');

% gyro block second:
cal3x4 = Rid*[gyroCalMatrix -gyroCalMatrix*gyroCalBiases];
vec = reshape(cal3x4, 12, 1); % JSON file stores the cal3x4 elements in column-wide order:

fprintf(fid, '  "gyroscope": {\n');
fprintf(fid, '    "%d": [\n', SensorTypeIdentifier);
for i=1:12
    fprintf(fid, '      %8.6f,\n', vec(i) );
end
fprintf(fid, '    ]\n');
fprintf(fid, '  },');


% magnetometer block third:
cal3x4 = [0 1 0 0; 0 0 -1 0; -1 0 0 0];
vec = reshape(cal3x4, 12, 1); % JSON file stores the cal3x4 elements in column-wide order:

fprintf(fid, '  "magnetometer": {\n');
fprintf(fid, '    "%d": [\n', SensorTypeIdentifier);
for i=1:12
    fprintf(fid, '      %8.6f,\n', vec(i) );
end
fprintf(fid, '');
fprintf(fid, '    ]\n');
fprintf(fid, '  }');
fprintf(fid, '}\n');

fclose(fid);

done = true;

== matlab function ImuCalibrator3Pass/MATLAB Function4 ==
  data: gyroCalBiases output; gyroCalMatrix output; dw input; Mgyr input; df input; Macc input; Ggyr input; gyroCalBiases input; gyroCalMatrix input; accelCalBiases input; accelCalMatrix input; gyroGsensMatrix input; accelCalBiases output; accelCalMatrix output; gyroGsensMatrix output
function [gyroCalBiases, gyroCalMatrix, accelCalBiases, accelCalMatrix,  gyroGsensMatrix] = updateCal3(dw, Mgyr, df, Macc, Ggyr, gyroCalBiases, gyroCalMatrix, accelCalBiases, accelCalMatrix,  gyroGsensMatrix)

    gyroCalBiases = gyroCalBiases + (eye(3)+Mgyr)*dw;
    gyroGsensMatrix = gyroGsensMatrix + (eye(3)+Mgyr)*Ggyr;
    gyroCalMatrix = inv(eye(3) + Mgyr) * gyroCalMatrix;

    accelCalBiases = accelCalBiases + df + Macc*df;
    accelCalMatrix =inv(eye(3) + Macc) * accelCalMatrix;

== matlab function ImuCalibrator3Pass/secondPass/MATLAB Function1 ==
  data: datarow output; EOF output
function [datarow, EOF] = readLineAscii()

persistent data data2 nrows row

if isempty(data)
    % row format = # SeqID, DeviceID, timestamp (sec), gyroXYZ (rad/sec), accelXYZ (m/s^2), temperature (degC)
    coder.varsize('data', [500000, 10], [1 0]);  % ten columns,  up to 200k rows
    data = load('imudata.txt', '-ascii'); 
    
    validTimestamp = data(:,3) > 0.001;
    data2 = data(validTimestamp, [4 5 6 7 8 9 3]); % select just the useful columns and rows
    nrows = size(data2, 1);
    row = 2;  % skip the first row since we need delta-t's

end

datarow = data2(row,:)';
datarow(7) = data2(row,7) - data2(row-1,7); % calculate Delta-t

EOF = row >= nrows;
row = row + 1;

== matlab function ImuCalibrator3Pass/thirdPass/MATLAB Function1 ==
  data: datarow output; EOF output
function [datarow, EOF] = readLineAscii()

persistent data data2 nrows row

if isempty(data)
    % row format = # SeqID, DeviceID, timestamp (sec), gyroXYZ (rad/sec), accelXYZ (m/s^2), temperature (degC)
    coder.varsize('data', [500000, 10], [1 0]);  % ten columns,  up to 200k rows
    data = load('imudata.txt', '-ascii'); 
    
    validTimestamp = data(:,3) > 0.001;
    data2 = data(validTimestamp, [4 5 6 7 8 9 3]); % select just the useful columns and rows
    nrows = size(data2, 1);
    row = 2;  % skip the first row since we need delta-t's

end

datarow = data2(row,:)';
datarow(7) = data2(row,7) - data2(row-1,7); % calculate Delta-t

EOF = row >= nrows;
row = row + 1;
